simulink model "Lab4PIIDD"  (R2018a)
settings: Solver=VariableStepAuto  StartTime=0.0  StopTime=15  RelTol=1e-3
undefined symbols (not defined in the file): kd, kd2, ki, ki2, kp
settings Model: Creator=Pc  LastModifiedBy=Pc
settings SolverCC: ZeroCrossAlgorithm=Adaptive
settings DebuggingCC: MaxConsecutiveZCsMsg=none

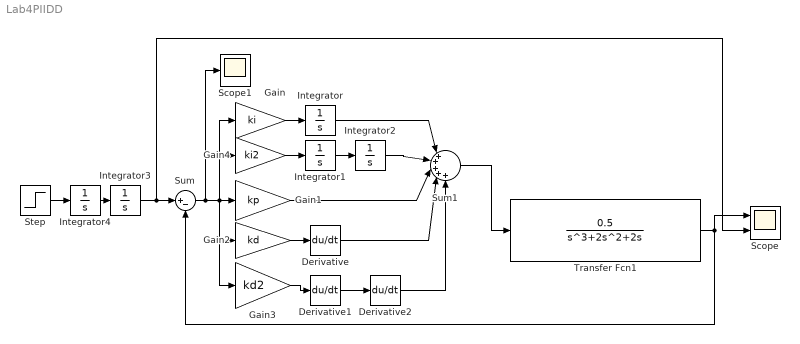
== system Lab4PIIDD ==
  Derivative : Derivative
  Derivative1 : Derivative
  Derivative2 : Derivative
  Gain : Gain  Gain=ki
  Gain1 : Gain  Gain=kp
  Gain2 : Gain  Gain=kd
  Gain3 : Gain  Gain=kd2
  Gain4 : Gain  Gain=ki2
  Integrator{,1..4} (5 alike) : Integrator
  Scope : Scope  NumInputPorts=2
  Scope1 : Scope
  Step : Step  SampleTime=0
  Sum : Sum  Inputs=|+-
  Sum1 : Sum  Inputs=|+++++
  Transfer Fcn1 : TransferFcn  Numerator=[0.5]  Denominator=[1 2 2 0]
  wires:
  Integrator/1 -> Sum1/1
  Gain2/1 -> Derivative/1
  Gain/1 -> Integrator/1
  Sum/1 -> Gain4/1, Gain/1, Gain1/1, Gain3/1, Gain2/1, Scope1/1
  Gain3/1 -> Derivative1/1
  Derivative1/1 -> Derivative2/1
  Transfer Fcn1/1 -> Scope/1, Sum/2
  Sum1/1 -> Transfer Fcn1/1
  Gain4/1 -> Integrator1/1
  Derivative2/1 -> Sum1/5
  Derivative/1 -> Sum1/4
  Gain1/1 -> Sum1/3
  Integrator1/1 -> Integrator2/1
  Integrator2/1 -> Sum1/2
  Integrator3/1 -> Scope/2, Sum/1
  Step/1 -> Integrator4/1
  Integrator4/1 -> Integrator3/1
